simulink model "postureRegulatorslx"  (R2023b)
settings: Solver=VariableStepAuto  StartTime=0.0  StopTime=100  RelTol=1e-3
libraries: robotmobilelib x1
settings Model: Creator=v4pal  LastModifiedBy=v4pal

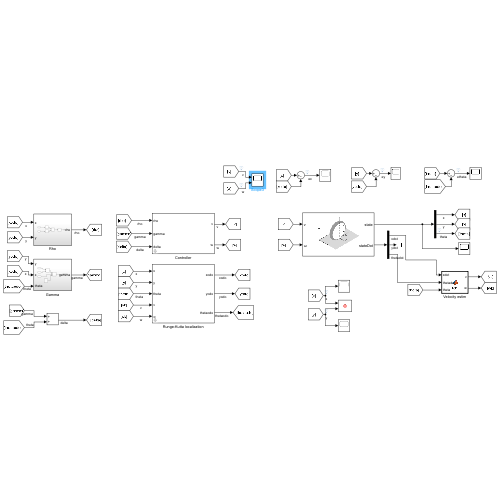
[thumbnail: Simulink's stored preview of the top-level diagram]
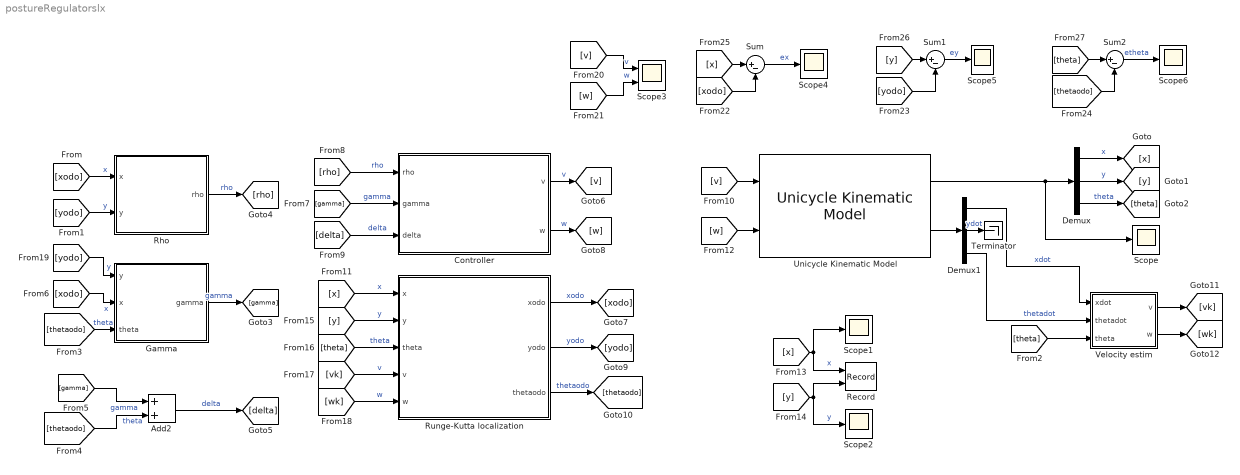
== system postureRegulatorslx ==
  Add2 : Sum
  Controller : Subsystem  mask{k1=0.25, k2=0.25, k3=0.25}
  Demux : Demux  Outputs=3
  Demux1 : Demux  Outputs=3
  Gamma : Subsystem
  Record : Record  FileSettingsInternal="{\"entries\":[{\"content\":{\"excelSettings\":{\"content\":{},\"type\":\"Streamout.ExcelSettings\"}},\"type\":\"Streamout.FileSettingStorage\",\"uuid\":\"\"}],\"packageUris\":[\"http:\\/\\/schema.mathworks.com\\/mf0\\/streamout_blocks\\/R2020a\"],\"version\":\"1.0\"}"  Layout=[1 1]  SignalsInternal="{\"entries\":[{\"content\":{\"signals\":[{\"content\":{\"blockPath\":[],\"dimensions\":[1],\"domain\":\"\",\"lineColor\":\"#d95319\",\"port\":1,\"sid\":[\"\"],\"signalID\":923,\"signalName\":\"x\"},\"type\":\"RecordBlkView.Signal\",\"uuid\":\"\"},{\"content\":{\"blockPath\":[],\"dimensions\":[1],\"domain\":\"\",\"lineColor\":\"#edb120\",\"port\":2,\"sid\":[\"\"],\"signalID\":927,\"signalName\":\"y\"},\"type\":\"RecordBlkView.Signal\",\"uuid\":\"\"}]},\"type\":\"RecordBlkView.InputSignals\",\"uuid\":\"\"}],\"packageUris\":[\"http:\\/\\/schema.mathworks.com\\/mf0\\/streamout_blocks\\/R2020a\"],\"version\":\"1.0\"}"  VisualizationBindings="{\"xyplotplugin\":{\"info\":[{\"series\":[],\"subplotID\":1}]}}"
  Rho : Subsystem
  Runge-Kutta localization : Subsystem  mask{Ts=0.05}
  Scope{,1..2,4..6} (6 alike) : Scope
  Scope3 : Scope  NumInputPorts=2
  Sum : Sum  Inputs=|+-
  Sum1 : Sum  Inputs=|+-
  Sum2 : Sum  Inputs=|+-
  Terminator : Terminator
  Unicycle Kinematic Model : robotmobilelib/Unicycle Kinematic Model  VehicleInputs=Vehicle Speed & Heading Angular Velocity  WheelRadius=0.1  WheelSpeedRange=[-Inf Inf]  InitialState=[1; 1; pi/4]  SimulateUsing=Interpreted execution
  Velocity estim : MATLAB Function  TreatAsAtomicUnit=on
  wires:
  Unicycle Kinematic Model/2 -> Demux1/1
  Demux/1 -> [x]  "x"
  Demux/2 -> [y]  "y"
  Demux/3 -> [theta]  "theta"
  [gamma] -> Add2/1  "gamma"
  [thetaodo] -> Add2/2  "theta"
  Add2/1 -> [delta]  "delta"
  [xodo] -> Rho/1(x)  "x"
  [yodo] -> Rho/2(y)  "y"
  [yodo] -> Gamma/1(y)  "y"
  [xodo] -> Gamma/2(x)  "x"
  [thetaodo] -> Gamma/3(theta)  "theta"
  Gamma/1(gamma) -> [gamma]  "gamma"
  Rho/1(rho) -> [rho]  "rho"
  [rho] -> Controller/1(rho)  "rho"
  [gamma] -> Controller/2(gamma)  "gamma"
  Controller/1(v) -> [v]  "v"
  [v] -> Unicycle Kinematic Model/1
  [w] -> Unicycle Kinematic Model/2
  [x] -> Record/1, Scope1/1  "x"
  [y] -> Record/2, Scope2/1  "y"
  Controller/2(w) -> [w]  "w"
  [delta] -> Controller/3(delta)  "delta"
  Unicycle Kinematic Model/1 -> Scope/1, Demux/1
  Demux1/1 -> Velocity estim/1(xdot)  "xdot"
  Velocity estim/1(v) -> [vk]
  Velocity estim/2(w) -> [wk]
  [theta] -> Velocity estim/3(theta)
  Demux1/3 -> Velocity estim/2(thetadot)  "thetadot"
  Demux1/2 -> Terminator/1  "ydot"
  [v] -> Scope3/1  "v"
  [w] -> Scope3/2  "w"
  [x] -> Sum/1
  [xodo] -> Sum/2
  [yodo] -> Sum1/2
  [y] -> Sum1/1
  Sum/1 -> Scope4/1  "ex"
  Sum1/1 -> Scope5/1  "ey"
  [theta] -> Sum2/1
  [thetaodo] -> Sum2/2
  Sum2/1 -> Scope6/1  "etheta"
  [x] -> Runge-Kutta localization/1(x)  "x"
  [y] -> Runge-Kutta localization/2(y)  "y"
  [theta] -> Runge-Kutta localization/3(theta)  "theta"
  [vk] -> Runge-Kutta localization/4(v)  "v"
  [wk] -> Runge-Kutta localization/5(w)  "w"
  Runge-Kutta localization/1(xodo) -> [xodo]  "xodo"
  Runge-Kutta localization/2(yodo) -> [yodo]  "yodo"
  Runge-Kutta localization/3(thetaodo) -> [thetaodo]  "thetaodo"

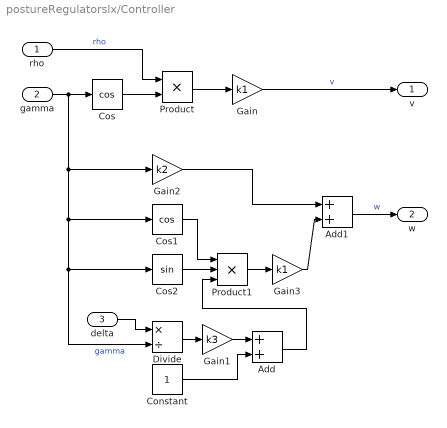
== system postureRegulatorslx/Controller ==
  rho : Inport
  gamma : Inport  Port=2
  delta : Inport  Port=3
  Add : Sum
  Add1 : Sum
  Constant : Constant
  Cos : Trigonometry  Operator=cos
  Cos1 : Trigonometry  Operator=cos
  Cos2 : Trigonometry
  Divide : Product  Inputs=*/
  Gain : Gain  Gain=k1
  Gain1 : Gain  Gain=k3
  Gain2 : Gain  Gain=k2
  Gain3 : Gain  Gain=k1
  Product : Product
  Product1 : Product  Inputs=3
  v : Outport
  w : Outport  Port=2
  wires:
  Product/1 -> Gain/1
  rho/1 -> Product/1  "rho"
  Cos/1 -> Product/2
  gamma/1 -> Cos/1, Divide/2, Cos2/1, Cos1/1, Gain2/1  "gamma"
  Gain/1 -> v/1  "v"
  Add1/1 -> w/1  "w"
  Gain1/1 -> Add/1
  delta/1 -> Divide/1
  Cos2/1 -> Product1/2
  Add/1 -> Product1/3
  Gain2/1 -> Add1/1
  Product1/1 -> Gain3/1
  Gain3/1 -> Add1/2
  Cos1/1 -> Product1/1
  Constant/1 -> Add/2
  Divide/1 -> Gain1/1

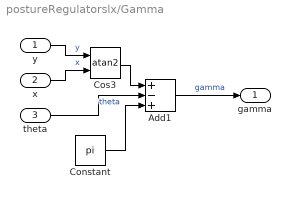
== system postureRegulatorslx/Gamma ==
  y : Inport
  x : Inport  Port=2
  theta : Inport  Port=3
  Add1 : Sum  Inputs=+-+
  Constant : Constant  Value=pi
  Cos3 : Trigonometry  Operator=atan2
  gamma : Outport
  wires:
  Cos3/1 -> Add1/1
  y/1 -> Cos3/1  "y"
  theta/1 -> Add1/2  "theta"
  x/1 -> Cos3/2  "x"
  Add1/1 -> gamma/1  "gamma"
  Constant/1 -> Add1/3

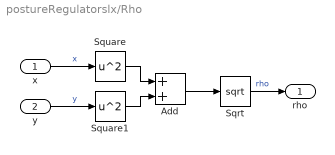
== system postureRegulatorslx/Rho ==
  x : Inport
  y : Inport  Port=2
  Add : Sum
  Sqrt : Sqrt
  Square : Math  Operator=square
  Square1 : Math  Operator=square
  rho : Outport
  wires:
  Add/1 -> Sqrt/1
  Square/1 -> Add/1
  x/1 -> Square/1  "x"
  Square1/1 -> Add/2
  y/1 -> Square1/1  "y"
  Sqrt/1 -> rho/1  "rho"

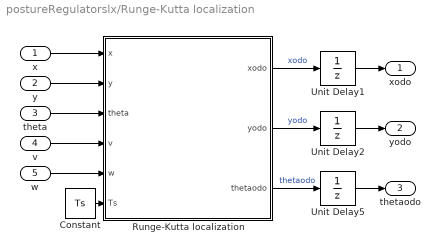
== system postureRegulatorslx/Runge-Kutta localization ==
  x : Inport
  y : Inport  Port=2
  theta : Inport  Port=3
  v : Inport  Port=4
  w : Inport  Port=5
  Constant : Constant  Value=Ts
  Runge-Kutta localization : MATLAB Function  TreatAsAtomicUnit=on
  Unit Delay1 : UnitDelay  InitialCondition=1  SampleTime=Ts  HasFrameUpgradeWarning=on
  Unit Delay2 : UnitDelay  InitialCondition=1  SampleTime=Ts  HasFrameUpgradeWarning=on
  Unit Delay5 : UnitDelay  InitialCondition=pi/4  SampleTime=Ts  HasFrameUpgradeWarning=on
  xodo : Outport
  yodo : Outport  Port=2
  thetaodo : Outport  Port=3
  wires:
  Constant/1 -> Runge-Kutta localization/6(Ts)
  Runge-Kutta localization/3(thetaodo) -> Unit Delay5/1  "thetaodo"
  theta/1 -> Runge-Kutta localization/3(theta)
  Unit Delay1/1 -> xodo/1
  Runge-Kutta localization/1(xodo) -> Unit Delay1/1  "xodo"
  Runge-Kutta localization/2(yodo) -> Unit Delay2/1  "yodo"
  v/1 -> Runge-Kutta localization/4(v)
  Unit Delay5/1 -> thetaodo/1
  Unit Delay2/1 -> yodo/1
  x/1 -> Runge-Kutta localization/1(x)
  w/1 -> Runge-Kutta localization/5(w)
  y/1 -> Runge-Kutta localization/2(y)

== matlab function postureRegulatorslx/Velocity estim ==
  data: xdot input; v output; thetadot input; theta input; w output
function [v, w] = fcn(xdot, thetadot, theta)

    % Computing velocities from the internal states 
    v = xdot / cos(theta);
    w = thetadot;

== matlab function postureRegulatorslx/Runge-Kutta localization/Runge-Kutta localization ==
  data: x input; xodo output; y input; theta input; v input; w input; Ts input; yodo output; thetaodo output
function [xodo, yodo, thetaodo] = localization(x,y,theta,v,w,Ts)

    % x(k+1)
    xodo = x + v * Ts * cos(theta + .5*w*Ts);
    % y(k+1)
    yodo = y + v * Ts * sin(theta + .5*w*Ts);
    % theta(k+1)
    thetaodo = theta + w*Ts;
